simulink model "DAC"  (R2024b)
settings: Solver=VariableStepAuto  StartTime=0.0  StopTime=1  RelTol=1e-3
libraries: dspstat3 x1
settings Model: Creator=s1920  LastModifiedBy=s1920

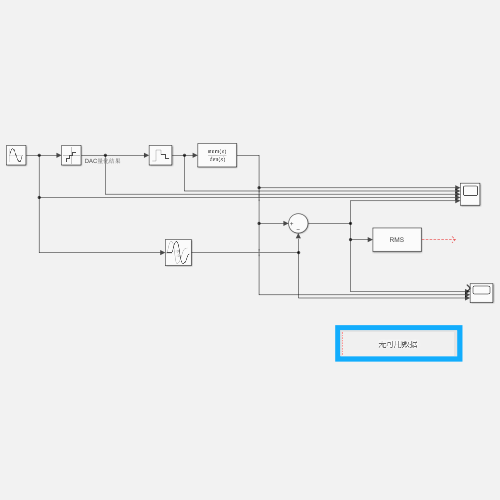
[thumbnail: Simulink's stored preview of the top-level diagram]
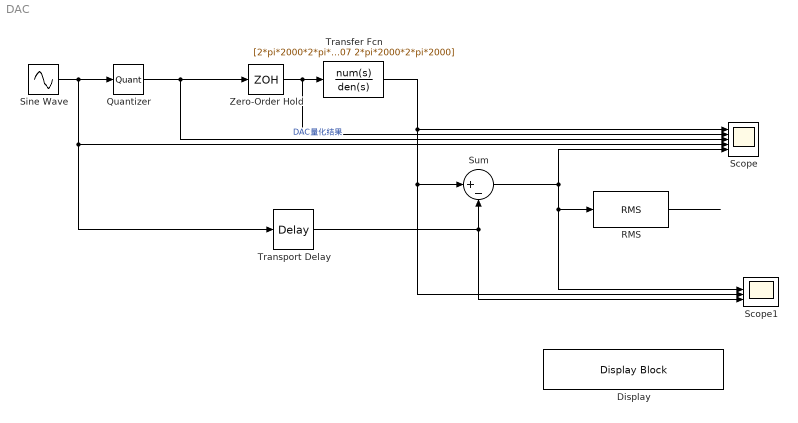
== system DAC ==
  Display : DisplayBlock  LabelPosition=Hide  Transparency=1
  Quantizer : Quantizer  QuantizationInterval=3.3/10
  RMS : dspstat3/RMS  run=off  directionMode=Each column  dimension=1  InputProcessing=Columns as channels (frame based)  reset_popup=None
  Scope : Scope  NumInputPorts=5
  Scope1 : Scope  NumInputPorts=4
  Sine Wave : Sin  Frequency=2*pi*1000  SampleTime=0
  Sum : Sum  Inputs=|+-
  Transfer Fcn : TransferFcn  Numerator=[2*pi*2000*2*pi*2000]  Denominator=[1 2*pi*2000/0.707 2*pi*2000*2*pi*2000]
  Transport Delay : TransportDelay  DelayTime=0.0001203
  Zero-Order Hold : ZeroOrderHold  SampleTime=1e-7
  wires:
  Sine Wave/1 -> Quantizer/1, Transport Delay/1, Scope/4
  Quantizer/1 -> Zero-Order Hold/1, Scope/3  "DAC量化结果"
  Zero-Order Hold/1 -> Scope/2, Transfer Fcn/1
  Transfer Fcn/1 -> Scope1/3, Sum/1, Scope/1
  Transport Delay/1 -> Scope1/4, Sum/2
  Sum/1 -> Scope1/2, RMS/1, Scope/5
  RMS/1 -> ?
